simulink model "lv_test7"  (Simulink 7.1)
settings: Solver=ode4  StartTime=0.0  StopTime=500  FixedStep=0.01  RelTol=1e-3
values from neighbouring files (symbols this model uses):
  C = abs(d-B)    [fuzzycontrol.m]    (also in lv_demofile6.m = 1450000)
  Jem = 90    [lv_cankaofile.m]    (also in lv_demofile.m = 97.5; lv_demofile1.m = 97.5; lv_demofile2.m = 97.5; lv_demofile3.m = 97.5)
  Jwt = 9e7    (= 90000000)    [lv_cankaofile.m]    (also in lv_demofile.m = 3275300; lv_demofile1.m = 3275300; lv_demofile2.m = 3275300; lv_demofile3.m = 3275300)
  K = 83    [lv_cankaofile.m]    (also in lv_demofile.m; lv_demofile1.m = 75.76; lv_demofile2.m; lv_demofile3.m = 75.76)
  R = 40    [lv_cankaofile.m]    (also in lv_demofile.m = 38.5; lv_demofile1.m = 38.75; lv_demofile2.m = 38.5; lv_demofile3.m = 38.5)
  ro_air = 1.225    [lv_cankaofile.m]    (also in lv_demofile.m = 1.2236; lv_demofile1.m; lv_demofile2.m = 1.2236; lv_demofile3.m)
libraries: simulink_extras x1, wt_blockset_v3 x1, simulink x1, DRlib x1
settings Model: Creator=lv  LastModifiedBy=lv

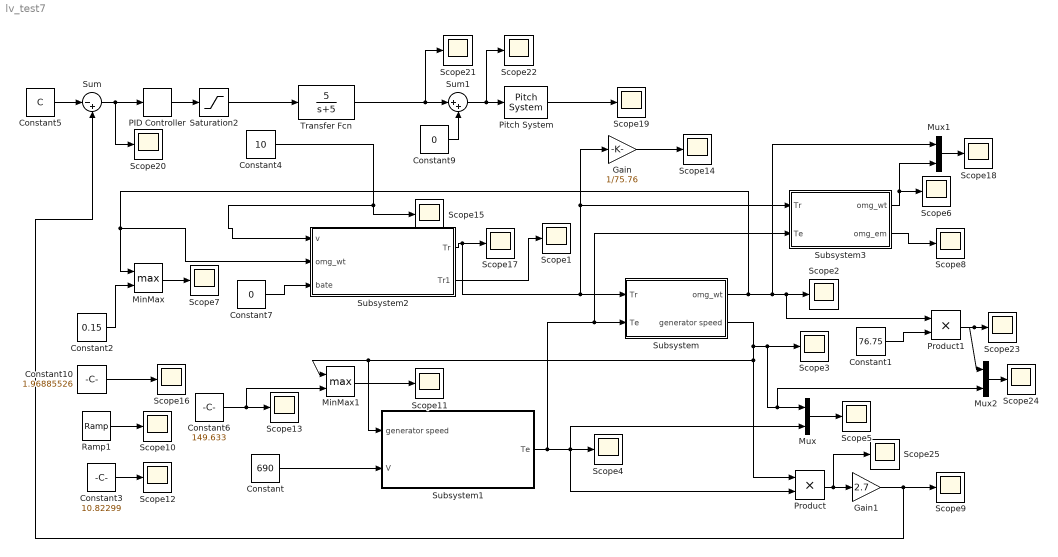
== system lv_test7 ==
  Constant : Constant  Value=690  OutDataType=sfix(16)  OutScaling=2^0
  Constant1 : Constant  Value=76.75  OutDataType=sfix(16)  OutScaling=2^0
  Constant10 : Constant  Value=1.96885526  OutDataType=sfix(16)  OutScaling=2^0
  Constant2 : Constant  Value=0.15  OutDataType=sfix(16)  OutScaling=2^0
  Constant3 : Constant  Value=10.82299  OutDataType=sfix(16)  OutScaling=2^0
  Constant4 : Constant  Value=10  OutDataType=sfix(16)  OutScaling=2^0
  Constant5 : Constant  Value=C  OutDataType=sfix(16)  OutScaling=2^0
  Constant6 : Constant  Value=149.633  OutDataType=sfix(16)  OutScaling=2^0
  Constant7 : Constant  Value=0  OutDataType=sfix(16)  OutScaling=2^0
  Constant9 : Constant  Value=0  OutDataType=sfix(16)  OutScaling=2^0
  Gain : Gain  Gain=1/75.76  ParameterDataType=sfix(16)  ParameterScaling=2^0  OutDataType=sfix(16)  OutScaling=2^0
  Gain1 : Gain  Gain=2.7  ParameterDataType=sfix(16)  ParameterScaling=2^0  OutDataType=sfix(16)  OutScaling=2^0
  MinMax : MinMax  Function=max  Inputs=2  OutDataType=sfix(16)  OutScaling=2^0
  MinMax1 : MinMax  Function=max  Inputs=2  OutDataType=sfix(16)  OutScaling=2^0
  Mux : Mux  Inputs=2
  Mux1 : Mux  Inputs=2
  Mux2 : Mux  Inputs=2
  PID Controller : simulink_extras/Additional Linear/PID Controller  SystemSampleTime=-1  P=5  I=1  D=0
  Pitch System : wt_blockset_v3/Control/WT Controller 2 MW DFIG/Pitch System  SystemSampleTime=-1
  Product : Product  OutDataType=sfix(16)  OutScaling=2^0  RndMeth=Zero
  Product1 : Product  OutDataType=sfix(16)  OutScaling=2^0  RndMeth=Zero
  Ramp1 : simulink/Sources/Ramp  SystemSampleTime=-1  slope=0.5  start=0  X0=0
  Saturation2 : Saturate  UpperLimit=inf  LowerLimit=1e-6  OutDataType=sfix(16)  OutScaling=2^0
  Scope{1..25} (25 alike) : Scope
      Scope1 settings: TimeRange=500  YMin=258138  YMax=285310
      Scope10 settings: TimeRange=12  YMin=-3e+010  YMax=5e+010  SaveName=ScopeData23
      Scope11 settings: TimeRange=12  YMin=78.5724  YMax=78.5724  SaveName=ScopeData34
      Scope12 settings: TimeRange=12  YMin=-3e+010  YMax=5e+010  SaveName=ScopeData27
      Scope13 settings: TimeRange=12  YMin=-3e+010  YMax=5e+010  SaveName=ScopeData28
      Scope14 settings: TimeRange=1000  YMin=8843.86  YMax=9774.8  SaveName=ScopeData29
      Scope15 settings: TimeRange=500  YMin=7.5  YMax=11.75  SaveName=ScopeData42
      Scope16 settings: TimeRange=12  YMin=-3e+010  YMax=5e+010  SaveName=ScopeData31
      Scope17 settings: TimeRange=500  YMin=406477  YMax=449264  SaveName=ScopeData32
      Scope18 settings: TimeRange=12  YMin=93  YMax=104  SaveName=ScopeData25
      Scope19 settings: YMin=9.5e-007  YMax=1.05e-006  SaveName=ScopeData36
      Scope2 settings: TimeRange=500  YMin=1.9685  YMax=1.971  SaveName=ScopeData2
      Scope20 settings: YMin=-153381  YMax=-138773  SaveName=ScopeData37
      Scope21 settings: YMin=9.5e-007  YMax=1.05e-006  SaveName=ScopeData38
      Scope22 settings: YMin=-2.25e+010  YMax=1.5e+010  SaveName=ScopeData35
      Scope23 settings: TimeRange=12  YMin=-2.46e+009  YMax=-2.36e+009  SaveName=ScopeData40
      Scope24 settings: TimeRange=12  YMin=78.5717  YMax=78.5717  SaveName=ScopeData41
      Scope25 settings: TimeRange=12  YMin=997500  YMax=1.0325e+006  SaveName=ScopeData43
      Scope3 settings: TimeRange=0.09310352246070133  YMin=123.4  YMax=124.7  SaveName=ScopeData3
      Scope4 settings: TimeRange=12  YMin=3450  YMax=4200  SaveName=ScopeData5
      Scope5 settings: TimeRange=12  YMin=0  YMax=2500  SaveName=ScopeData17
      Scope6 settings: TimeRange=500  YMin=25  YMax=110  SaveName=ScopeData19
      Scope7 settings: TimeRange=12  YMin=-3e+010  YMax=5e+010  SaveName=ScopeData18
      Scope8 settings: TimeRange=500  YMin=920207  YMax=920207  SaveName=ScopeData24
      Scope9 settings: TimeRange=12  YMin=1.52398e+006  YMax=1.52398e+006  SaveName=ScopeData22
  Subsystem : Subsystem
  Subsystem1 : Subsystem
  Subsystem2 : Subsystem
  Subsystem3 : Subsystem
  Sum : Sum  Inputs=|-+  OutDataType=sfix(16)  OutScaling=2^0  SaturateOnIntegerOverflow=on
  Sum1 : Sum  Inputs=|++  OutDataType=sfix(16)  OutScaling=2^0  SaturateOnIntegerOverflow=on
  Transfer Fcn : TransferFcn  Numerator=[5]  Denominator=[1 5]
  wires:
  Subsystem/1(omg_wt) -> Mux1/1, Scope2/1, Product1/1, MinMax/1, Subsystem2/2(omg_wt)
  Subsystem/2(generator speed) -> Scope3/1, Mux/1, Mux2/2, Product/1, MinMax1/1, Subsystem1/1(generator speed)
  Constant/1 -> Subsystem1/2(V)
  Subsystem1/1(Te) -> Scope4/1, Product/2, Mux/2, Subsystem/2(Te), Subsystem3/2(Te)
  Ramp1/1 -> Scope10/1
  Constant2/1 -> MinMax/2
  Mux/1 -> Scope5/1
  MinMax/1 -> Scope7/1
  Constant3/1 -> Scope12/1
  Constant6/1 -> Scope13/1, MinMax1/2
  Gain/1 -> Scope14/1
  Constant10/1 -> Scope16/1
  Subsystem2/1(Tr) -> Scope17/1, Subsystem/1(Tr), Gain/1, Subsystem3/1(Tr)
  Subsystem3/1(omg_wt) -> Scope6/1, Mux1/2
  Subsystem3/2(omg_em) -> Scope8/1
  Mux1/1 -> Scope18/1
  MinMax1/1 -> Scope11/1
  Sum/1 -> PID Controller/1, Scope20/1
  Constant5/1 -> Sum/1
  PID Controller/1 -> Saturation2/1
  Saturation2/1 -> Transfer Fcn/1
  Pitch System/1 -> Scope19/1
  Transfer Fcn/1 -> Sum1/1, Scope21/1
  Sum1/1 -> Pitch System/1, Scope22/1
  Constant9/1 -> Sum1/2
  Constant1/1 -> Product1/2
  Product1/1 -> Scope23/1, Mux2/1
  Mux2/1 -> Scope24/1
  Constant4/1 -> Subsystem2/1(v), Scope15/1
  Subsystem2/2(Tr1) -> Scope1/1
  Product/1 -> Gain1/1, Scope25/1
  Gain1/1 -> Scope9/1, Sum/2
  Constant7/1 -> Subsystem2/3(bate)

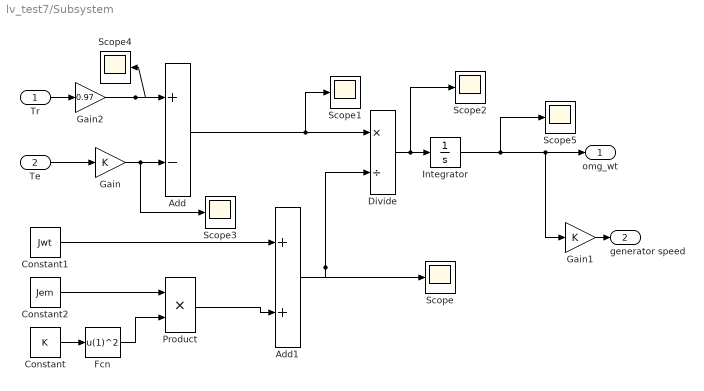
== system lv_test7/Subsystem ==
  Tr : Inport  OutDataType=sfix(16)  OutScaling=2^0
  Te : Inport  Port=2  OutDataType=sfix(16)  OutScaling=2^0
  Add : Sum  Inputs=+-  OutDataType=sfix(16)  OutScaling=2^-10
  Add1 : Sum  OutDataType=sfix(16)  OutScaling=2^-10
  Constant : Constant  Value=K  OutDataType=sfix(16)  OutScaling=2^0
  Constant1 : Constant  Value=Jwt  OutDataType=sfix(16)  OutScaling=2^0
  Constant2 : Constant  Value=Jem  OutDataType=sfix(16)  OutScaling=2^0
  Divide : Product  Inputs=*/  OutDataType=sfix(16)  OutScaling=2^-10
  Fcn : Fcn  Expr=u(1)^2
  Gain : Gain  Gain=K  ParameterDataType=sfix(16)  ParameterScaling=2^0  OutDataType=sfix(16)  OutScaling=2^0
  Gain1 : Gain  Gain=K  ParameterDataType=sfix(16)  ParameterScaling=2^0  OutDataType=sfix(16)  OutScaling=2^0
  Gain2 : Gain  Gain=0.97  ParameterDataType=sfix(16)  ParameterScaling=2^0  OutDataType=sfix(16)  OutScaling=2^0
  Integrator : Integrator  InitialCondition=1.96885526  UpperSaturationLimit=2.3
  Product : Product  OutDataType=sfix(16)  OutScaling=2^0  RndMeth=Zero
  Scope{,1..5} (6 alike) : Scope
      Scope settings: SaveName=ScopeData5
      Scope1 settings: SaveName=ScopeData6
      Scope2 settings: SaveName=ScopeData7
      Scope3 settings: SaveName=ScopeData26
      Scope4 settings: SaveName=ScopeData39
      Scope5 settings: YMin=3.80274  YMax=3.80274  SaveName=ScopeData30
  omg_wt : Outport  OutDataType=sfix(16)  OutScaling=2^0
  generator speed : Outport  Port=2  OutDataType=sfix(16)  OutScaling=2^0
  wires:
  Gain1/1 -> generator speed/1
  Divide/1 -> Integrator/1, Scope2/1
  Add1/1 -> Divide/2, Scope/1
  Add/1 -> Divide/1, Scope1/1
  Product/1 -> Add1/2
  Constant1/1 -> Add1/1
  Constant2/1 -> Product/1
  Gain/1 -> Add/2, Scope3/1
  Te/1 -> Gain/1
  Constant/1 -> Fcn/1
  Fcn/1 -> Product/2
  Integrator/1 -> omg_wt/1, Gain1/1, Scope5/1
  Tr/1 -> Gain2/1
  Gain2/1 -> Add/1, Scope4/1

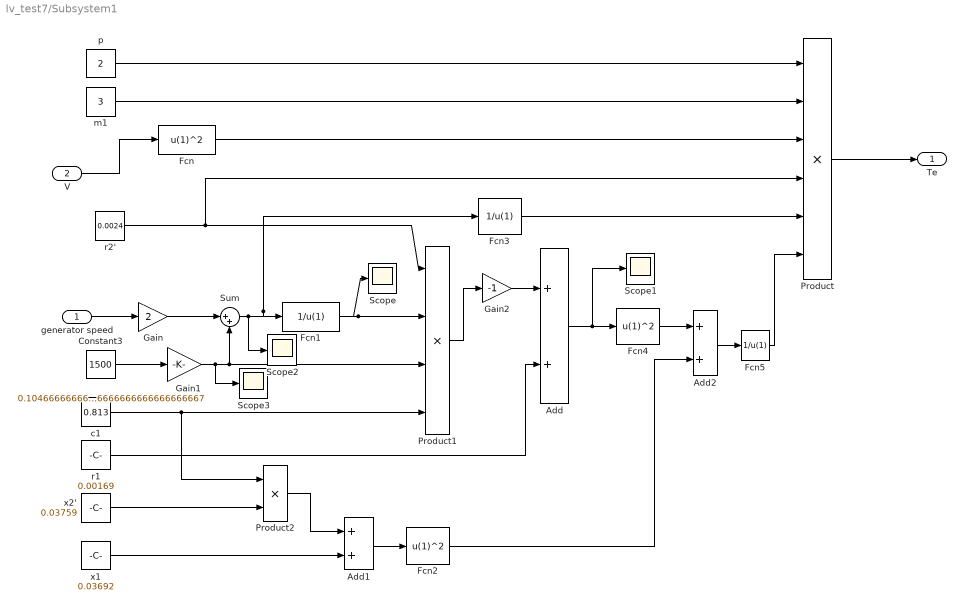
== system lv_test7/Subsystem1 ==
  generator speed : Inport  OutDataType=sfix(16)  OutScaling=2^0
  V : Inport  Port=2  OutDataType=sfix(16)  OutScaling=2^0
  Add : Sum  OutDataType=sfix(16)  OutScaling=2^-10
  Add1 : Sum  OutDataType=sfix(16)  OutScaling=2^-10
  Add2 : Sum  OutDataType=sfix(16)  OutScaling=2^-10
  Constant3 : Constant  Value=1500  OutDataType=sfix(16)  OutScaling=2^0
  Fcn : Fcn  Expr=u(1)^2
  Fcn1 : Fcn  Expr=1/u(1)
  Fcn2 : Fcn  Expr=u(1)^2
  Fcn3 : Fcn  Expr=1/u(1)
  Fcn4 : Fcn  Expr=u(1)^2
  Fcn5 : Fcn  Expr=1/u(1)
  Gain : Gain  Gain=2  ParameterDataType=sfix(16)  ParameterScaling=2^0  OutDataType=sfix(16)  OutScaling=2^0
  Gain1 : Gain  Gain=0.10466666666666666666666666666667  ParameterDataType=sfix(16)  ParameterScaling=2^0  OutDataType=sfix(16)  OutScaling=2^0
  Gain2 : Gain  Gain=-1  ParameterDataType=sfix(16)  ParameterScaling=2^0  OutDataType=sfix(16)  OutScaling=2^0
  Product : Product  Inputs=6  OutDataType=sfix(16)  OutScaling=2^0  RndMeth=Zero
  Product1 : Product  Inputs=4  OutDataType=sfix(16)  OutScaling=2^0  RndMeth=Zero
  Product2 : Product  OutDataType=sfix(16)  OutScaling=2^0  RndMeth=Zero
  Scope{,1..3} (4 alike) : Scope
      Scope settings: YMin=0  YMax=100000  SaveName=ScopeData10
      Scope1 settings: YMin=0  YMax=100000  SaveName=ScopeData11
      Scope2 settings: YMin=0  YMax=100000  SaveName=ScopeData15
      Scope3 settings: YMin=0  YMax=100000  SaveName=ScopeData9
  Sum : Sum  Inputs=|++  OutDataType=sfix(16)  OutScaling=2^0
  c1 : Constant  Value=0.813  OutDataType=sfix(16)  OutScaling=2^0
  m1 : Constant  Value=3  OutDataType=sfix(16)  OutScaling=2^0
  p : Constant  Value=2  OutDataType=sfix(16)  OutScaling=2^0
  r1 : Constant  Value=0.00169  OutDataType=sfix(16)  OutScaling=2^0
  r2' : Constant  Value=0.0024  OutDataType=sfix(16)  OutScaling=2^0
  x1 : Constant  Value=0.03692  OutDataType=sfix(16)  OutScaling=2^0
  x2' : Constant  Value=0.03759  OutDataType=sfix(16)  OutScaling=2^0
  Te : Outport  OutDataType=sfix(16)  OutScaling=2^0
  wires:
  Fcn1/1 -> Scope/1, Product1/2
  Product/1 -> Te/1
  Fcn5/1 -> Product/6
  Add2/1 -> Fcn5/1
  Fcn2/1 -> Add2/2
  Fcn4/1 -> Add2/1
  Add/1 -> Scope1/1, Fcn4/1
  Fcn3/1 -> Product/5
  Gain2/1 -> Add/1
  r1/1 -> Add/2
  Fcn/1 -> Product/3
  m1/1 -> Product/2
  p/1 -> Product/1
  Product1/1 -> Gain2/1
  Add1/1 -> Fcn2/1
  x1/1 -> Add1/2
  Product2/1 -> Add1/1
  x2'/1 -> Product2/2
  c1/1 -> Product2/1, Product1/4
  r2'/1 -> Product/4, Product1/1
  Sum/1 -> Scope2/1, Fcn1/1, Fcn3/1
  Gain1/1 -> Product1/3, Sum/2, Scope3/1
  Constant3/1 -> Gain1/1
  Gain/1 -> Sum/1
  generator speed/1 -> Gain/1
  V/1 -> Fcn/1

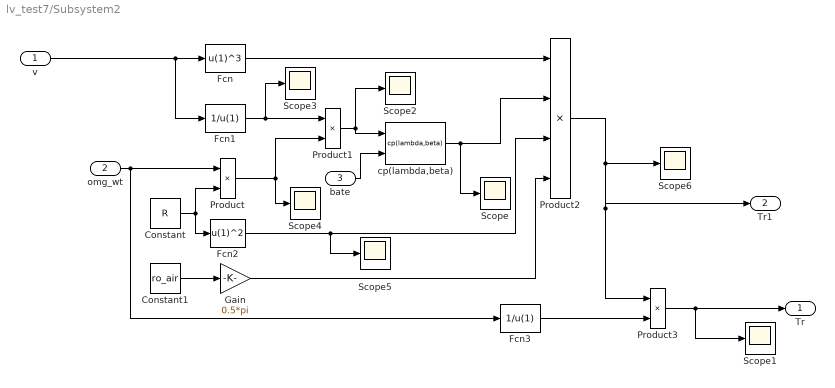
== system lv_test7/Subsystem2 ==
  v : Inport  OutDataType=sfix(16)  OutScaling=2^0
  omg_wt : Inport  Port=2  OutDataType=sfix(16)  OutScaling=2^0
  bate : Inport  Port=3  OutDataType=sfix(16)  OutScaling=2^0
  Constant : Constant  Value=R  OutDataType=sfix(16)  OutScaling=2^0
  Constant1 : Constant  Value=ro_air  OutDataType=sfix(16)  OutScaling=2^0
  Fcn : Fcn  Expr=u(1)^3
  Fcn1 : Fcn  Expr=1/u(1)
  Fcn2 : Fcn  Expr=u(1)^2
  Fcn3 : Fcn  Expr=1/u(1)
  Gain : Gain  Gain=0.5*pi  ParameterDataType=sfix(16)  ParameterScaling=2^0  OutDataType=sfix(16)  OutScaling=2^0
  Product : Product  OutDataType=sfix(16)  OutScaling=2^0  RndMeth=Zero
  Product1 : Product  OutDataType=sfix(16)  OutScaling=2^0  RndMeth=Zero
  Product2 : Product  Inputs=4  OutDataType=sfix(16)  OutScaling=2^0  RndMeth=Zero
  Product3 : Product  OutDataType=sfix(16)  OutScaling=2^0  RndMeth=Zero
  Scope{,1..6} (7 alike) : Scope
      Scope settings: TimeRange=50  YMin=0.1772981595092024  YMax=0.2028981595092024  SaveName=ScopeData4
      Scope1 settings: TimeRange=20  YMin=-1500000  YMax=1500000
      Scope2 settings: SaveName=ScopeData6
      Scope3 settings: SaveName=ScopeData7
      Scope4 settings: SaveName=ScopeData8
      Scope5 settings: YMin=1426.48  YMax=1576.64  SaveName=ScopeData20
      Scope6 settings: TimeRange=20  YMin=-500000  YMax=5e+006  SaveName=ScopeData21
  cp(lambda,beta) : DRlib/Wind Generation/Wind Turbine/cp(lambda,beta)  SystemSampleTime=-1
  Tr : Outport  OutDataType=sfix(16)  OutScaling=2^0
  Tr1 : Outport  Port=2  OutDataType=sfix(16)  OutScaling=2^0
  wires:
  v/1 -> Fcn/1, Fcn1/1
  omg_wt/1 -> Product/1, Fcn3/1
  Constant/1 -> Product/2, Fcn2/1
  Fcn1/1 -> Product1/1, Scope3/1
  Product/1 -> Product1/2, Scope4/1
  Product1/1 -> Scope2/1, cp(lambda,beta)/1
  bate/1 -> cp(lambda,beta)/2
  Fcn/1 -> Product2/1
  cp(lambda,beta)/1 -> Product2/2, Scope/1
  Fcn2/1 -> Product2/3, Scope5/1
  Gain/1 -> Product2/4
  Constant1/1 -> Gain/1
  Product2/1 -> Scope6/1, Product3/1, Tr1/1
  Fcn3/1 -> Product3/2
  Product3/1 -> Scope1/1, Tr/1

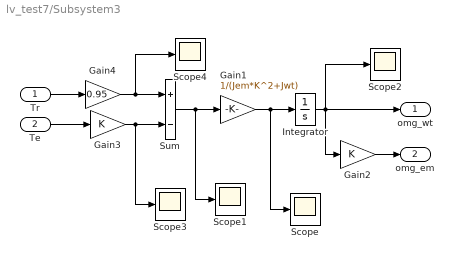
== system lv_test7/Subsystem3 ==
  Tr : Inport  OutDataType=sfix(16)  OutScaling=2^0
  Te : Inport  Port=2  OutDataType=sfix(16)  OutScaling=2^0
  Gain1 : Gain  Gain=1/(Jem*K^2+Jwt)  ParameterDataType=sfix(16)  ParameterScaling=2^0  OutDataType=sfix(16)  OutScaling=2^0  SaturateOnIntegerOverflow=on  OutDataTypeStr=Inherit: Same as input  ParamDataTypeStr=Inherit: Same as input
  Gain2 : Gain  Gain=K  ParameterDataType=sfix(16)  ParameterScaling=2^0  OutDataType=sfix(16)  OutScaling=2^0  SaturateOnIntegerOverflow=on  OutDataTypeStr=Inherit: Same as input  ParamDataTypeStr=Inherit: Same as input
  Gain3 : Gain  Gain=K  ParameterDataType=sfix(16)  ParameterScaling=2^0  OutDataType=sfix(16)  OutScaling=2^0  SaturateOnIntegerOverflow=on  OutDataTypeStr=Inherit: Same as input  ParamDataTypeStr=Inherit: Same as input
  Gain4 : Gain  Gain=0.95  ParameterDataType=sfix(16)  ParameterScaling=2^0  OutDataType=sfix(16)  OutScaling=2^0  SaturateOnIntegerOverflow=on  OutDataTypeStr=Inherit: Same as input  ParamDataTypeStr=Inherit: Same as input
  Integrator : Integrator  InitialCondition=2.07  UpperSaturationLimit=2.3  LowerSaturationLimit=0
  Scope{,1..4} (5 alike) : Scope
      Scope settings: YMin=0.00797839  YMax=0.00881823  SaveName=ScopeData12
      Scope1 settings: YMin=3361.62  YMax=3715.48  SaveName=ScopeData13
      Scope2 settings: YMin=1.03647  YMax=1.03647  SaveName=ScopeData14
      Scope3 settings: YMin=2.37692e+006  YMax=2.37692e+006  SaveName=ScopeData16
      Scope4 settings: YMin=892600  YMax=892600  SaveName=ScopeData33
  Sum : Sum  Inputs=+-  OutDataType=sfix(16)  OutScaling=2^0  SaturateOnIntegerOverflow=on  InputSameDT=on  OutDataTypeStr=Inherit: Same as first input
  omg_wt : Outport  OutDataType=sfix(16)  OutScaling=2^0  InitialOutput=0
  omg_em : Outport  Port=2  OutDataType=sfix(16)  OutScaling=2^0  InitialOutput=0
  wires:
  Gain1/1 -> Integrator/1, Scope/1
  Sum/1 -> Gain1/1, Scope1/1
  Te/1 -> Gain3/1
  Gain2/1 -> omg_em/1
  Gain3/1 -> Sum/2, Scope3/1
  Integrator/1 -> omg_wt/1, Gain2/1, Scope2/1
  Tr/1 -> Gain4/1
  Gain4/1 -> Sum/1, Scope4/1
